simulink model "read_control"  (R2020a)
settings: Solver=FixedStepDiscrete  StartTime=0.0  StopTime=10.0  RelTol=1e-3
settings Model: Creator=thomas  LastModifiedBy=thomas

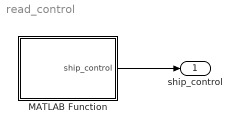
== system read_control ==
  MATLAB Function : MATLAB Function  TreatAsAtomicUnit=on
  ship_control : Outport  OutDataTypeStr=Bus: ShipControl
  wires:
  MATLAB Function/1(ship_control) -> ship_control/1

== matlab function read_control/MATLAB Function ==
  data: ship_control output Bus: ShipControl
function ship_control =read_control
    coder.extrinsic('evalin');
    ship_control.pitch = 0.0;
    ship_control.yaw = 0.0;
    ship_control.roll = 0.0;
    ship_control.pitch = evalin('base', 'vessel_control.getPitch();');
    ship_control.yaw = evalin('base', 'vessel_control.getYaw();');
    ship_control.roll = evalin('base', 'vessel_control.getRoll();');
    
end
